simulink model "DCMotorSpeedControl_OpenLoop"  (R2015b)
settings: Solver=VariableStepAuto  StartTime=0.0  StopTime=1  RelTol=1e-3
values from neighbouring files (symbols this model uses):
  Kv = (Vdc_nom - (I_nl*R_winding))/Om_nl    (= 0.00375385553259)    [MotorModel_Mabuchi_RS_540.m]    (also in Params.m = 0.0039)
  Vdc = 9.6    [MotorModel_Mabuchi_RS_540.m]    (also in Params.m)
libraries: LocalLib x2
settings Model: Creator=jje  LastModifiedBy=jje

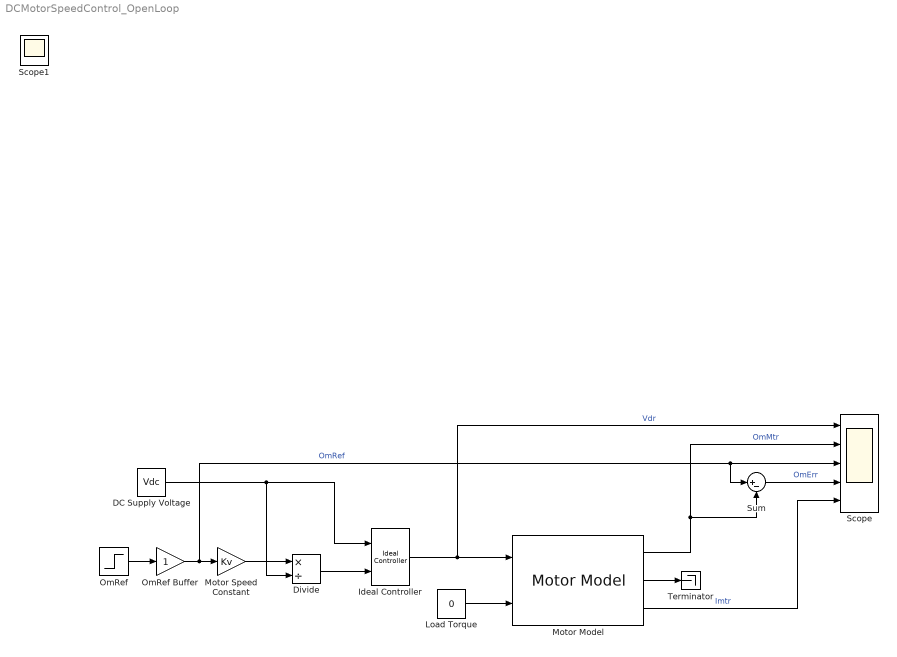
== system DCMotorSpeedControl_OpenLoop ==
  DC Supply Voltage : Constant  Value=Vdc
  Divide : Product  Inputs=*/
  Ideal Controller : LocalLib/Ideal Controller
  Load Torque : Constant  Value=0
  Motor Model : LocalLib/Motor Model
  Motor Speed Constant : Gain  Gain=Kv
  OmRef : Step  Time=0.01  After=20000*2*pi/60  SampleTime=0
  OmRef Buffer : Gain
  Scope : Scope  NumInputPorts=5
  Sum : Sum  Inputs=|+-
  Terminator : Terminator
  Scope1 : Scope
  wires:
  DC Supply Voltage/1 -> Divide/2, Ideal Controller/1
  Ideal Controller/1 -> Motor Model/1, Scope/1  "Vdr"
  Motor Model/1 -> Sum/2, Scope/2  "OmMtr"
  Load Torque/1 -> Motor Model/2
  OmRef/1 -> OmRef Buffer/1
  OmRef Buffer/1 -> Sum/1, Scope/3, Motor Speed Constant/1  "OmRef"
  Motor Speed Constant/1 -> Divide/1
  Divide/1 -> Ideal Controller/2
  Sum/1 -> Scope/4  "OmErr"
  Motor Model/3 -> Scope/5  "Imtr"
  Motor Model/2 -> Terminator/1
